simulink model "Simulink_file_newversion"  (R2024a)
settings: Solver=VariableStepAuto  StartTime=0.0  StopTime=5  RelTol=1e-3
values from neighbouring files (symbols this model uses):
  DG = cell(1, numOfDGs)    [evaluateDesigns.m]
  K = cell(1, numDGs)    [Centralized_Controller_For_DG.m]    (also in Centralized_Controller_For_DG_with_Constraints.m; ComputePassivityForDGs.m = sdpvar(1, 3, 'full'); GetPassivityForDGs.m = sdpvar(1, 3, 'full'); Global_Controller_Synthesis.m = cell(N, N))
  Line = cell(1, numOfLines)    [evaluateDesigns.m]
  V_ref = 48    [Global_Controller_Synthesis.m]
undefined symbols (not defined in the file or in its folder): ChangeGlobalLoad1, ChangeGlobalLoad2, PlugIn, PlugOut, R_Global, V_nom
libraries: spsSeriesRLCBranchLib x26, spsCurrentMeasurementLib x8, spsVoltageMeasurementLib x5, simulink x4, spsDCVoltageSourceLib x4, spsDiodeLib x4, spsIGBTLib x4, spsIdealSwitchLib x2, spsStairGeneratorLib x2, spspowerguiLib x1
settings Model: Creator=najaf  LastModifiedBy=najaf
settings RTWCC: GPUComputeCapability=3.5

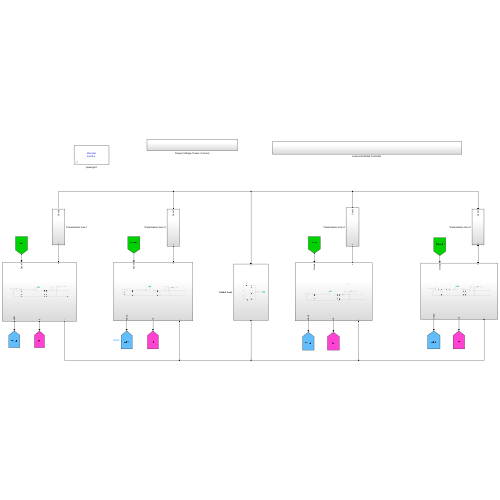
[thumbnail: Simulink's stored preview of the top-level diagram]
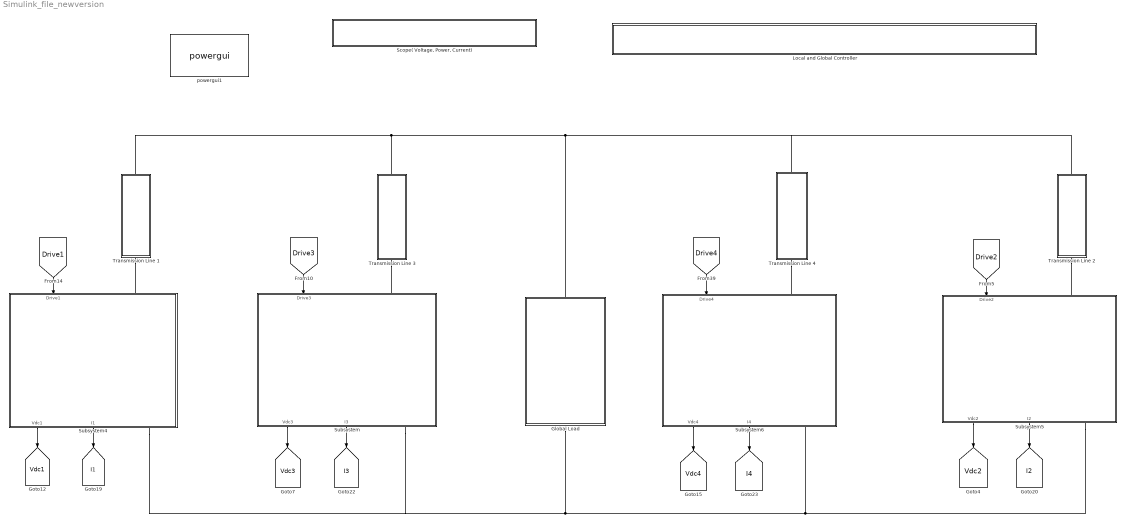
== system Simulink_file_newversion ==
  Global Load : Subsystem
  "Local and Global Controller " : Subsystem
  "Scope( Voltage, Power, Current)" : Subsystem
  Subsystem : Subsystem
      settings: PortSchema="{\"entries\":[{\"content\":{\"sides\":[{\"content\":{},\"type\":\"ConnectorPlacement.EquallySpacedRectSide\",\"uuid\":\"08b51d35-5d4f-4d5f-a5b0-37344ba45088\"},{\"content\":{\"side\":\"RIGHT\"},\"type\":\"ConnectorPlacement.EquallySpacedRectSide\",\"uuid\":\"3324977a-6e34-487c-ade0-88e1bff4bebb\"},{\"content\":{\"connectorIds\":[\"In1\",\"LConn1\"],\"side\":\"TOP\"},\"type\":\"ConnectorPlacement.EquallySpacedRectSide\",\"uuid\":\"e322db0d-0a35-4471-b922-f546e4cab97b\"},{\"content\":{\"connectorIds\":[\"Out1\",\"Out2\",\"RConn1\"],\"side\":\"BOTTOM\"},\"type\":\"ConnectorPlacement.EquallySpacedRectSide\",\"uuid\":\"57a428a6-4844-4d68-bda7-c5e0dfb814f7\"}]},\"type\":\"ConnectorPlacement.EquallySpacedConnector\",\"uuid\":\"93cb8cb8-3b8c-4430-b1f3-cf7722d9fa22\"}],\"packageUris\":[\"http://schema.mathworks.com/mf0/Connector/R2020b\"],\"version\":\"1.0\"}"
  Subsystem4 : Subsystem
      settings: PortSchema="{\"entries\":[{\"content\":{\"sides\":[{\"content\":{},\"type\":\"ConnectorPlacement.EquallySpacedRectSide\",\"uuid\":\"764b3ce9-8ebc-4171-9263-333df0dfe6fc\"},{\"content\":{\"side\":\"RIGHT\"},\"type\":\"ConnectorPlacement.EquallySpacedRectSide\",\"uuid\":\"c1e9d8a4-dae3-47b0-883a-539aeb69869c\"},{\"content\":{\"connectorIds\":[\"In1\",\"LConn1\"],\"side\":\"TOP\"},\"type\":\"ConnectorPlacement.EquallySpacedRectSide\",\"uuid\":\"bcad0197-72c7-4543-a9ab-ea7942b9cd59\"},{\"content\":{\"connectorIds\":[\"Out1\",\"Out2\",\"RConn1\"],\"side\":\"BOTTOM\"},\"type\":\"ConnectorPlacement.EquallySpacedRectSide\",\"uuid\":\"beb0f75b-103e-4e06-b52f-abd8ae36630a\"}]},\"type\":\"ConnectorPlacement.EquallySpacedConnector\",\"uuid\":\"3998def4-aed0-48b8-bc2a-5ab2d5ec9fd3\"}],\"packageUris\":[\"http://schema.mathworks.com/mf0/Connector/R2020b\"],\"version\":\"1.0\"}"
  Subsystem5 : Subsystem
      settings: PortSchema="{\"entries\":[{\"content\":{\"sides\":[{\"content\":{},\"type\":\"ConnectorPlacement.EquallySpacedRectSide\",\"uuid\":\"08b51d35-5d4f-4d5f-a5b0-37344ba45088\"},{\"content\":{\"side\":\"RIGHT\"},\"type\":\"ConnectorPlacement.EquallySpacedRectSide\",\"uuid\":\"3324977a-6e34-487c-ade0-88e1bff4bebb\"},{\"content\":{\"connectorIds\":[\"In1\",\"LConn1\"],\"side\":\"TOP\"},\"type\":\"ConnectorPlacement.EquallySpacedRectSide\",\"uuid\":\"e322db0d-0a35-4471-b922-f546e4cab97b\"},{\"content\":{\"connectorIds\":[\"Out1\",\"Out2\",\"RConn1\"],\"side\":\"BOTTOM\"},\"type\":\"ConnectorPlacement.EquallySpacedRectSide\",\"uuid\":\"f52eba1b-ac2a-4c74-a10c-8b92ab05ae45\"}]},\"type\":\"ConnectorPlacement.EquallySpacedConnector\",\"uuid\":\"93cb8cb8-3b8c-4430-b1f3-cf7722d9fa22\"}],\"packageUris\":[\"http://schema.mathworks.com/mf0/Connector/R2020b\"],\"version\":\"1.0\"}"
  Subsystem6 : Subsystem
      settings: PortSchema="{\"entries\":[{\"content\":{\"sides\":[{\"content\":{},\"type\":\"ConnectorPlacement.EquallySpacedRectSide\",\"uuid\":\"764b3ce9-8ebc-4171-9263-333df0dfe6fc\"},{\"content\":{\"side\":\"RIGHT\"},\"type\":\"ConnectorPlacement.EquallySpacedRectSide\",\"uuid\":\"c1e9d8a4-dae3-47b0-883a-539aeb69869c\"},{\"content\":{\"connectorIds\":[\"In1\",\"LConn1\"],\"side\":\"TOP\"},\"type\":\"ConnectorPlacement.EquallySpacedRectSide\",\"uuid\":\"bcad0197-72c7-4543-a9ab-ea7942b9cd59\"},{\"content\":{\"connectorIds\":[\"Out1\",\"Out2\",\"RConn1\"],\"side\":\"BOTTOM\"},\"type\":\"ConnectorPlacement.EquallySpacedRectSide\",\"uuid\":\"43195860-d6e2-4bd9-a504-1cc2264ea7f4\"}]},\"type\":\"ConnectorPlacement.EquallySpacedConnector\",\"uuid\":\"3998def4-aed0-48b8-bc2a-5ab2d5ec9fd3\"}],\"packageUris\":[\"http://schema.mathworks.com/mf0/Connector/R2020b\"],\"version\":\"1.0\"}"
  Transmission Line 1 : Subsystem
  Transmission Line 2 : Subsystem
  Transmission Line 3 : Subsystem
  Transmission Line 4 : Subsystem
  powergui1 : spspowerguiLib/powergui  Priority=1  SimulationMode=Discrete  SampleTime=2e-5  frequency=60  Iterations=50  frequencyindice=0  Pbase=100e6  ErrMax=1e-4  UnitsV=kV  UnitsW=MW  buscounter=0  FunctionMessages=off  echomessages=off  EnableUseOfTLC=off  CurrentSourceSwitches=off  DisableSnubberDevices=off  DisableRonSwitches=off  DisableVfSwitches=off  DisplayEquations=off  AutomaticDiscreteSolvers=off  SolverType=Tustin/Backward Euler (TBE)  Interpol=off  ExternalGateDelay=off  methode=off  Ts=100  x0status=blocks  SPID=on  SwTol=0  HookPort=off  NonlinearTolerance=1e-4  nMaxIteration=100  ContinueOnMaxIteration=off  RestoreLinks=warning  ResistiveCurrentMeasurement=off  Frange=[0:2:500]  Ylog=off  Xlog=on  ShowGrid=off  save=off  variable=ZData  structure=0  ZoomFFT=off  StartTime=0.0  cycles=1  DisplayStyle=1  fundamental=60  FreqAxis=off  MaxFrequency=1000  frequencyindicesteady=1  RmsSteady=1  display=off
  tag scope: I1=global, I2=global, I3=global, I4=global, Vdc1=global, Vdc2=global, Vdc3=global, Vdc4=global
  wires:
  [Drive4] -> Subsystem6/1(Drive4)
  Subsystem6/1(Vdc4) -> [Vdc4]
  Subsystem6/2(I4) -> [I4]
  [Drive1] -> Subsystem4/1(Drive1)
  Subsystem4/1(Vdc1) -> [Vdc1]
  Subsystem4/2(I1) -> [I1]
  [Drive2] -> Subsystem5/1(Drive2)
  [Drive3] -> Subsystem/1(Drive3)
  Subsystem/2(I3) -> [I3]
  Subsystem/1(Vdc3) -> [Vdc3]
  Subsystem5/1(Vdc2) -> [Vdc2]
  Subsystem5/2(I2) -> [I2]
  connections:
  Transmission Line 1/LConn1 -- Subsystem4/LConn1
  Subsystem5/RConn1 -- Subsystem4/RConn1 -- Subsystem/RConn1 -- Global Load/RConn1 -- Subsystem6/RConn1
  Transmission Line 2/RConn1 -- Subsystem5/LConn1
  Transmission Line 3/RConn1 -- Subsystem/LConn1
  Transmission Line 4/RConn1 -- Subsystem6/LConn1
  Transmission Line 1/RConn1 -- Transmission Line 2/LConn1 -- Transmission Line 4/LConn1 -- Global Load/LConn1 -- Transmission Line 3/LConn1

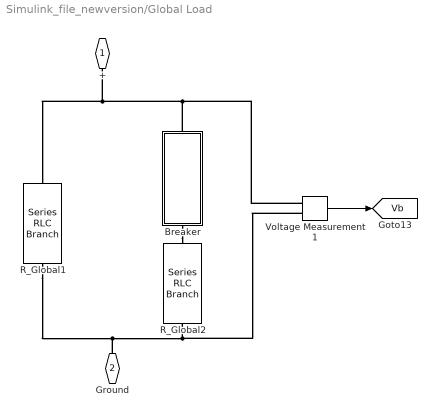
== system Simulink_file_newversion/Global Load ==
  Breaker : Subsystem
  R_Global1 : spsSeriesRLCBranchLib/Series RLC Branch  LConnTagsString=__new0  RConnTagsString=__new0  BranchType=R  Resistance=R_Global  Inductance=1e-3  SetiL0=off  InitialCurrent=0  Capacitance=1e-6  Setx0=off  InitialVoltage=0  Measurements=None
  R_Global2 : spsSeriesRLCBranchLib/Series RLC Branch  LConnTagsString=__new0  RConnTagsString=__new0  BranchType=R  Resistance=R_Global  Inductance=1e-3  SetiL0=off  InitialCurrent=0  Capacitance=1e-6  Setx0=off  InitialVoltage=0  Measurements=None
  Voltage Measurement1 : spsVoltageMeasurementLib/Voltage Measurement  PhasorSimulation=off  OutputType=Complex  PSBequivalent=0
  + : PMIOPort  Side=Left
  Ground : PMIOPort  Port=2  Side=Right
  tag scope: Vb=global
  wires:
  Voltage Measurement1/1 -> [Vb]
  connections:
  Ground/RConn1 -- Voltage Measurement1/LConn2 -- R_Global2/RConn1 -- R_Global1/RConn1
  Breaker/LConn1 -- R_Global1/LConn1 -- +/RConn1 -- Voltage Measurement1/LConn1
  Breaker/RConn1 -- R_Global2/LConn1

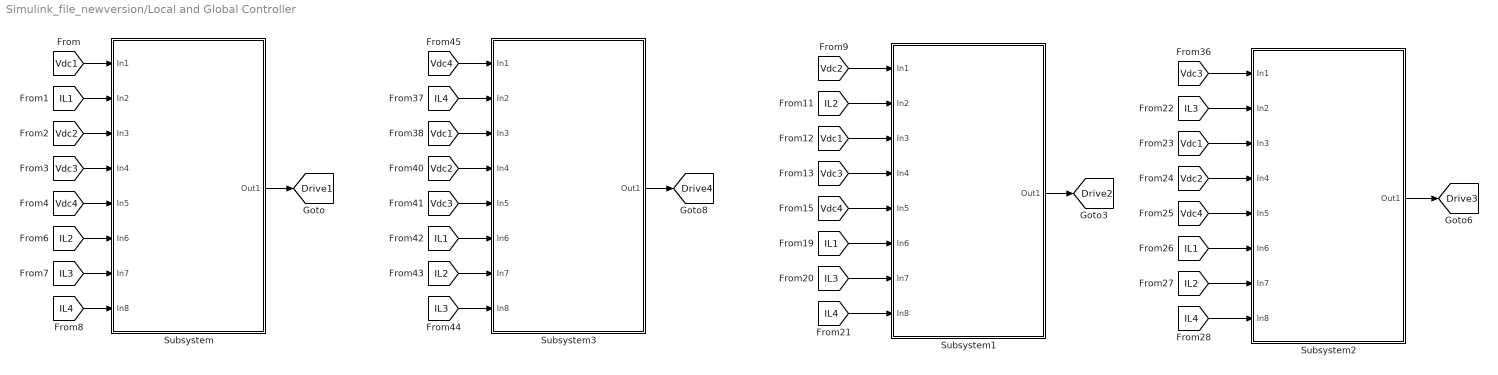
== system Simulink_file_newversion/Local and Global Controller  ==
  Subsystem : Subsystem
  Subsystem1 : Subsystem
  Subsystem2 : Subsystem
  Subsystem3 : Subsystem
  tag scope: Drive1=global, Drive2=global, Drive3=global, Drive4=global
  wires:
  [IL3] -> Subsystem3/8(In8)
  Subsystem3/1(Out1) -> [Drive4]
  [IL1] -> Subsystem3/6(In6)
  [IL2] -> Subsystem3/7(In7)
  [Vdc3] -> Subsystem1/4(In4)
  [IL4] -> Subsystem1/8(In8)
  [Vdc3] -> Subsystem3/5(In5)
  [IL4] -> Subsystem3/2(In2)
  [Vdc4] -> Subsystem3/1(In1)
  [Vdc1] -> Subsystem1/3(In3)
  [Vdc2] -> Subsystem3/4(In4)
  [Vdc1] -> Subsystem3/3(In3)
  [IL1] -> Subsystem1/6(In6)
  [Vdc4] -> Subsystem1/5(In5)
  [Vdc2] -> Subsystem1/1(In1)
  [IL3] -> Subsystem1/7(In7)
  Subsystem1/1(Out1) -> [Drive2]
  [IL2] -> Subsystem1/2(In2)
  Subsystem2/1(Out1) -> [Drive3]
  [IL3] -> Subsystem2/2(In2)
  [IL4] -> Subsystem2/8(In8)
  [Vdc2] -> Subsystem2/4(In4)
  [Vdc4] -> Subsystem2/5(In5)
  [IL1] -> Subsystem2/6(In6)
  [Vdc3] -> Subsystem2/1(In1)
  [Vdc1] -> Subsystem2/3(In3)
  [IL2] -> Subsystem2/7(In7)
  [Vdc2] -> Subsystem/3(In3)
  [Vdc4] -> Subsystem/5(In5)
  Subsystem/1(Out1) -> [Drive1]
  [IL2] -> Subsystem/6(In6)
  [IL3] -> Subsystem/7(In7)
  [IL4] -> Subsystem/8(In8)
  [IL1] -> Subsystem/2(In2)
  [Vdc1] -> Subsystem/1(In1)
  [Vdc3] -> Subsystem/4(In4)

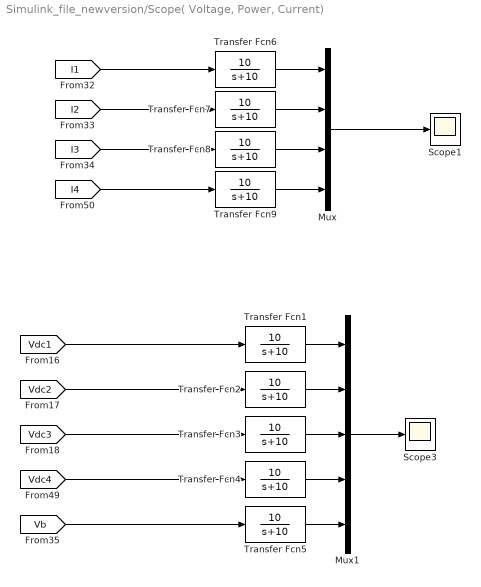
== system Simulink_file_newversion/Scope( Voltage, Power, Current) ==
  Mux : Mux
  Mux1 : Mux  Inputs=5
  Scope1 : Scope
  Scope3 : Scope
  Transfer Fcn{1..9} (9 alike) : TransferFcn  Numerator=[10]  Denominator=[1 10]
  wires:
  [I3] -> Transfer Fcn8/1
  [I2] -> Transfer Fcn7/1
  [I1] -> Transfer Fcn6/1
  Mux/1 -> Scope1/1
  [I4] -> Transfer Fcn9/1
  Mux1/1 -> Scope3/1
  [Vdc1] -> Transfer Fcn1/1
  [Vdc2] -> Transfer Fcn2/1
  [Vdc3] -> Transfer Fcn3/1
  [Vdc4] -> Transfer Fcn4/1
  [Vb] -> Transfer Fcn5/1
  Transfer Fcn1/1 -> Mux1/1
  Transfer Fcn2/1 -> Mux1/2
  Transfer Fcn3/1 -> Mux1/3
  Transfer Fcn4/1 -> Mux1/4
  Transfer Fcn5/1 -> Mux1/5
  Transfer Fcn6/1 -> Mux/1
  Transfer Fcn7/1 -> Mux/2
  Transfer Fcn8/1 -> Mux/3
  Transfer Fcn9/1 -> Mux/4

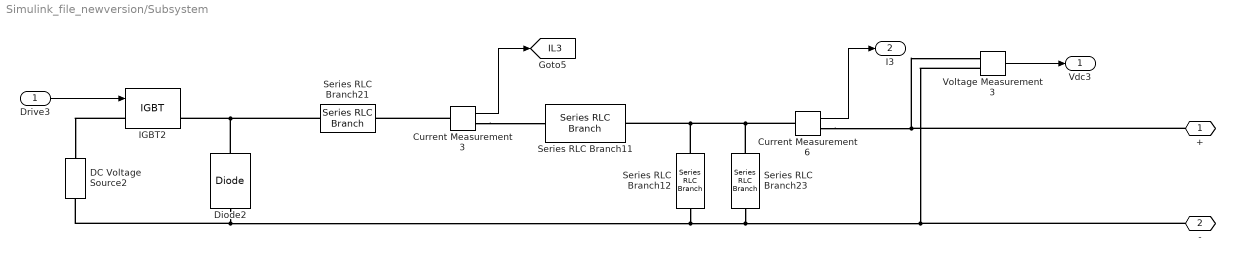
== system Simulink_file_newversion/Subsystem ==
  Drive3 : Inport
  Current Measurement3 : spsCurrentMeasurementLib/Current Measurement  PhasorSimulation=off  OutputType=Complex  PSBequivalent=0
  Current Measurement6 : spsCurrentMeasurementLib/Current Measurement  PhasorSimulation=off  OutputType=Complex  PSBequivalent=0
  DC Voltage Source2 : spsDCVoltageSourceLib/DC Voltage Source  Amplitude=V_nom  Measurements=None
  Diode2 : spsDiodeLib/Diode  Ron=0.001  Lon=0  Vf=0.8  IC=0  UseSnubber=off  Rs=500  Cs=0  Measurements=off
  IGBT2 : spsIGBTLib/IGBT  Ron=0.001  Lon=0  Vf=1  Tf=1e-6  Tt=2e-6  IC=0  Rs=1e5  Cs=inf  Measurements=on
  Series RLC Branch11 : spsSeriesRLCBranchLib/Series RLC Branch  LConnTagsString=__new0  RConnTagsString=__new0  BranchType=L  Resistance=1  Inductance=DG{3}.L  SetiL0=off  InitialCurrent=0  Capacitance=1e-6  Setx0=off  InitialVoltage=0  Measurements=Branch current
  Series RLC Branch12 : spsSeriesRLCBranchLib/Series RLC Branch  LConnTagsString=__new0  RConnTagsString=__new0  BranchType=C  Resistance=1  Inductance=1e-2  SetiL0=off  InitialCurrent=0  Capacitance=DG{3}.C  Setx0=off  InitialVoltage=0  Measurements=None
  Series RLC Branch21 : spsSeriesRLCBranchLib/Series RLC Branch  LConnTagsString=__new0  RConnTagsString=__new0  BranchType=R  Resistance=DG{3}.R  Inductance=1e-2  SetiL0=off  InitialCurrent=0  Capacitance=2.2e-3  Setx0=off  InitialVoltage=0  Measurements=None
  Series RLC Branch23 : spsSeriesRLCBranchLib/Series RLC Branch  LConnTagsString=__new0  RConnTagsString=__new0  BranchType=R  Resistance=DG{3}.Y  Inductance=1e-2  SetiL0=off  InitialCurrent=0  Capacitance=2.2e-3  Setx0=off  InitialVoltage=0  Measurements=None
  Voltage Measurement3 : spsVoltageMeasurementLib/Voltage Measurement  PhasorSimulation=off  OutputType=Complex  PSBequivalent=0
  + : PMIOPort  Side=Left
  - : PMIOPort  Port=2  Side=Right
  Vdc3 : Outport
  I3 : Outport  Port=2
  tag scope: IL3=global
  wires:
  Current Measurement3/1 -> [IL3]
  Drive3/1 -> IGBT2/1
  Current Measurement6/1 -> I3/1
  Voltage Measurement3/1 -> Vdc3/1
  connections:
  Series RLC Branch12/LConn1 -- Series RLC Branch23/LConn1 -- Current Measurement6/LConn1 -- Series RLC Branch11/RConn1
  Voltage Measurement3/LConn2 -- -/RConn1 -- Diode2/LConn1 -- DC Voltage Source2/LConn1 -- Series RLC Branch12/RConn1 -- Series RLC Branch23/RConn1
  Current Measurement6/RConn1 -- +/RConn1 -- Voltage Measurement3/LConn1
  Current Measurement3/LConn1 -- Series RLC Branch21/LConn1
  Current Measurement3/RConn1 -- Series RLC Branch11/LConn1
  Diode2/RConn1 -- Series RLC Branch21/RConn1 -- IGBT2/RConn1
  IGBT2/LConn1 -- DC Voltage Source2/RConn1

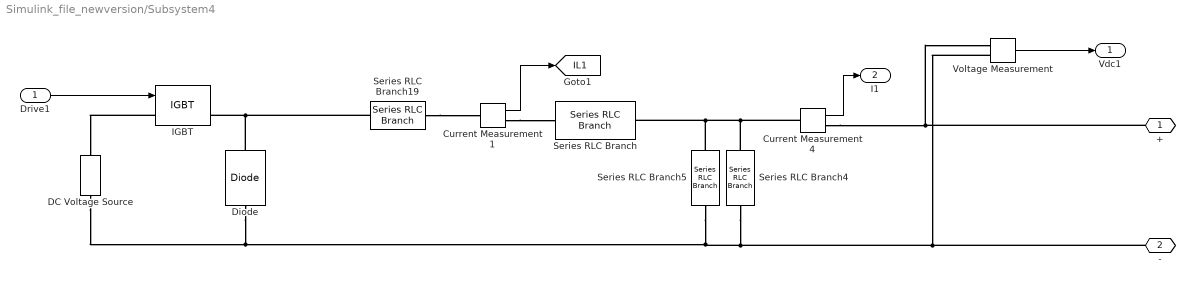
== system Simulink_file_newversion/Subsystem4 ==
  Drive1 : Inport
  Current Measurement1 : spsCurrentMeasurementLib/Current Measurement  PhasorSimulation=off  OutputType=Complex  PSBequivalent=0
  Current Measurement4 : spsCurrentMeasurementLib/Current Measurement  PhasorSimulation=off  OutputType=Complex  PSBequivalent=0
  DC Voltage Source : spsDCVoltageSourceLib/DC Voltage Source  Amplitude=V_nom  Measurements=None
  Diode : spsDiodeLib/Diode  Ron=0.001  Lon=0  Vf=0.8  IC=0  UseSnubber=off  Rs=500  Cs=0  Measurements=off
  IGBT : spsIGBTLib/IGBT  Ron=0.001  Lon=0  Vf=1  Tf=1e-6  Tt=2e-6  IC=0  Rs=1e5  Cs=inf  Measurements=on
  Series RLC Branch : spsSeriesRLCBranchLib/Series RLC Branch  LConnTagsString=__new0  RConnTagsString=__new0  BranchType=L  Resistance=1  Inductance=DG{1}.L  SetiL0=off  InitialCurrent=0  Capacitance=1e-6  Setx0=off  InitialVoltage=0  Measurements=Branch current
  Series RLC Branch19 : spsSeriesRLCBranchLib/Series RLC Branch  LConnTagsString=__new0  RConnTagsString=__new0  BranchType=R  Resistance=DG{1}.R  Inductance=1e-2  SetiL0=off  InitialCurrent=0  Capacitance=2.2e-3  Setx0=off  InitialVoltage=0  Measurements=None
  Series RLC Branch4 : spsSeriesRLCBranchLib/Series RLC Branch  LConnTagsString=__new0  RConnTagsString=__new0  BranchType=R  Resistance=DG{1}.Y  Inductance=1e-2  SetiL0=off  InitialCurrent=0  Capacitance=2.2e-3  Setx0=off  InitialVoltage=0  Measurements=None
  Series RLC Branch5 : spsSeriesRLCBranchLib/Series RLC Branch  LConnTagsString=__new0  RConnTagsString=__new0  BranchType=C  Resistance=1  Inductance=1e-2  SetiL0=off  InitialCurrent=0  Capacitance=DG{1}.C  Setx0=off  InitialVoltage=0  Measurements=None
  Voltage Measurement : spsVoltageMeasurementLib/Voltage Measurement  PhasorSimulation=off  OutputType=Complex  PSBequivalent=0
  + : PMIOPort  Side=Left
  - : PMIOPort  Port=2  Side=Right
  Vdc1 : Outport
  I1 : Outport  Port=2
  tag scope: IL1=global
  wires:
  Current Measurement1/1 -> [IL1]
  Current Measurement4/1 -> I1/1
  Voltage Measurement/1 -> Vdc1/1
  Drive1/1 -> IGBT/1
  connections:
  Current Measurement4/RConn1 -- +/RConn1 -- Voltage Measurement/LConn1
  Series RLC Branch4/RConn1 -- Voltage Measurement/LConn2 -- -/RConn1 -- DC Voltage Source/LConn1 -- Diode/LConn1 -- Series RLC Branch5/RConn1
  Series RLC Branch5/LConn1 -- Current Measurement4/LConn1 -- Series RLC Branch4/LConn1 -- Series RLC Branch/RConn1
  Current Measurement1/RConn1 -- Series RLC Branch/LConn1
  IGBT/LConn1 -- DC Voltage Source/RConn1
  Series RLC Branch19/LConn1 -- Current Measurement1/LConn1
  Diode/RConn1 -- Series RLC Branch19/RConn1 -- IGBT/RConn1

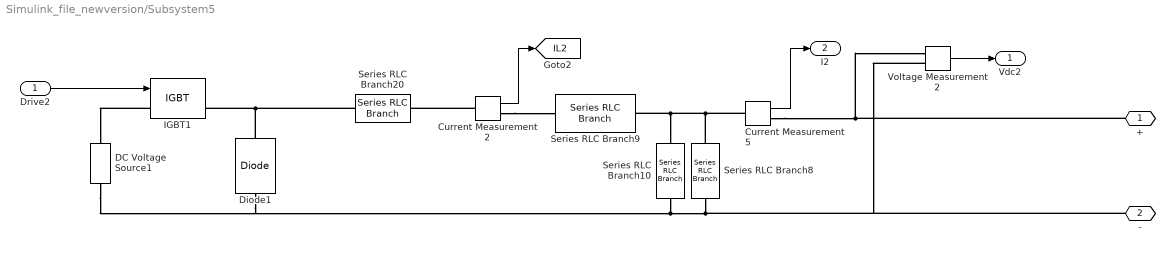
== system Simulink_file_newversion/Subsystem5 ==
  Drive2 : Inport
  Current Measurement2 : spsCurrentMeasurementLib/Current Measurement  PhasorSimulation=off  OutputType=Complex  PSBequivalent=0
  Current Measurement5 : spsCurrentMeasurementLib/Current Measurement  PhasorSimulation=off  OutputType=Complex  PSBequivalent=0
  DC Voltage Source1 : spsDCVoltageSourceLib/DC Voltage Source  Amplitude=V_nom  Measurements=None
  Diode1 : spsDiodeLib/Diode  Ron=0.001  Lon=0  Vf=0.8  IC=0  UseSnubber=off  Rs=500  Cs=0  Measurements=off
  IGBT1 : spsIGBTLib/IGBT  Ron=0.001  Lon=0  Vf=1  Tf=1e-6  Tt=2e-6  IC=0  Rs=1e5  Cs=inf  Measurements=on
  Series RLC Branch10 : spsSeriesRLCBranchLib/Series RLC Branch  LConnTagsString=__new0  RConnTagsString=__new0  BranchType=C  Resistance=1  Inductance=1e-2  SetiL0=off  InitialCurrent=0  Capacitance=DG{2}.C  Setx0=off  InitialVoltage=0  Measurements=None
  Series RLC Branch20 : spsSeriesRLCBranchLib/Series RLC Branch  LConnTagsString=__new0  RConnTagsString=__new0  BranchType=R  Resistance=DG{2}.R  Inductance=1e-2  SetiL0=off  InitialCurrent=0  Capacitance=2.2e-3  Setx0=off  InitialVoltage=0  Measurements=None
  Series RLC Branch8 : spsSeriesRLCBranchLib/Series RLC Branch  LConnTagsString=__new0  RConnTagsString=__new0  BranchType=R  Resistance=DG{2}.Y  Inductance=1e-2  SetiL0=off  InitialCurrent=0  Capacitance=2.2e-3  Setx0=off  InitialVoltage=0  Measurements=None
  Series RLC Branch9 : spsSeriesRLCBranchLib/Series RLC Branch  LConnTagsString=__new0  RConnTagsString=__new0  BranchType=L  Resistance=1  Inductance=DG{2}.L  SetiL0=off  InitialCurrent=0  Capacitance=1e-6  Setx0=off  InitialVoltage=0  Measurements=Branch current
  Voltage Measurement2 : spsVoltageMeasurementLib/Voltage Measurement  PhasorSimulation=off  OutputType=Complex  PSBequivalent=0
  + : PMIOPort  Side=Left
  - : PMIOPort  Port=2  Side=Right
  Vdc2 : Outport
  I2 : Outport  Port=2
  tag scope: IL2=global
  wires:
  Current Measurement2/1 -> [IL2]
  Drive2/1 -> IGBT1/1
  Current Measurement5/1 -> I2/1
  Voltage Measurement2/1 -> Vdc2/1
  connections:
  Series RLC Branch8/LConn1 -- Current Measurement5/LConn1 -- Series RLC Branch10/LConn1 -- Series RLC Branch9/RConn1
  Current Measurement5/RConn1 -- +/RConn1 -- Voltage Measurement2/LConn1
  Diode1/RConn1 -- Series RLC Branch20/RConn1 -- IGBT1/RConn1
  Series RLC Branch10/RConn1 -- DC Voltage Source1/LConn1 -- Diode1/LConn1 -- Voltage Measurement2/LConn2 -- -/RConn1 -- Series RLC Branch8/RConn1
  Current Measurement2/RConn1 -- Series RLC Branch9/LConn1
  Current Measurement2/LConn1 -- Series RLC Branch20/LConn1
  IGBT1/LConn1 -- DC Voltage Source1/RConn1

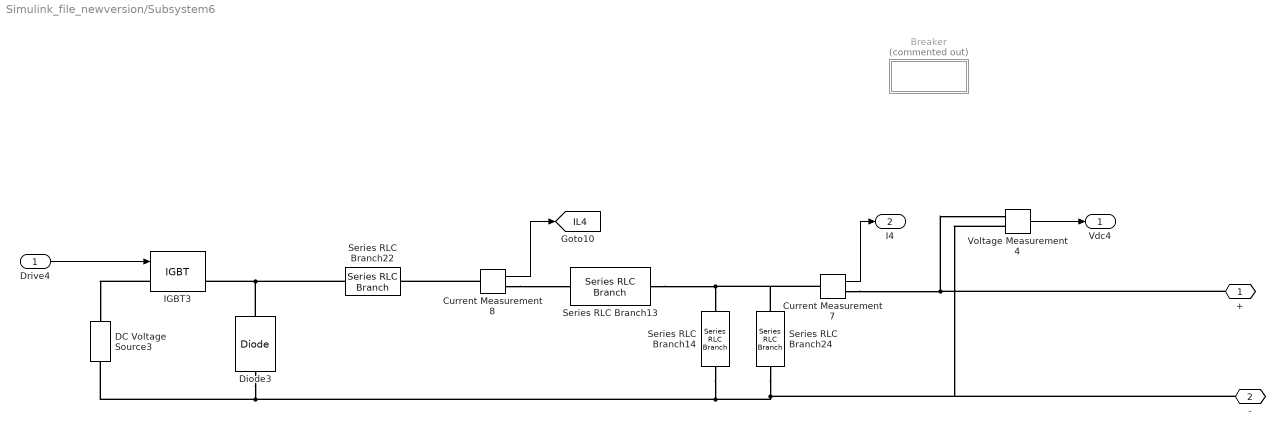
== system Simulink_file_newversion/Subsystem6 ==
  Drive4 : Inport
  Breaker : Subsystem  Commented=on
  Current Measurement7 : spsCurrentMeasurementLib/Current Measurement  PhasorSimulation=off  OutputType=Complex  PSBequivalent=0
  Current Measurement8 : spsCurrentMeasurementLib/Current Measurement  PhasorSimulation=off  OutputType=Complex  PSBequivalent=0
  DC Voltage Source3 : spsDCVoltageSourceLib/DC Voltage Source  Amplitude=V_nom  Measurements=None
  Diode3 : spsDiodeLib/Diode  Ron=0.001  Lon=0  Vf=0.8  IC=0  UseSnubber=off  Rs=500  Cs=0  Measurements=off
  IGBT3 : spsIGBTLib/IGBT  Ron=0.001  Lon=0  Vf=1  Tf=1e-6  Tt=2e-6  IC=0  Rs=1e5  Cs=inf  Measurements=on
  Series RLC Branch13 : spsSeriesRLCBranchLib/Series RLC Branch  LConnTagsString=__new0  RConnTagsString=__new0  BranchType=L  Resistance=1  Inductance=DG{4}.L  SetiL0=off  InitialCurrent=0  Capacitance=1e-6  Setx0=off  InitialVoltage=0  Measurements=Branch current
  Series RLC Branch14 : spsSeriesRLCBranchLib/Series RLC Branch  LConnTagsString=__new0  RConnTagsString=__new0  BranchType=C  Resistance=1  Inductance=1e-2  SetiL0=off  InitialCurrent=0  Capacitance=DG{4}.C  Setx0=off  InitialVoltage=0  Measurements=None
  Series RLC Branch22 : spsSeriesRLCBranchLib/Series RLC Branch  LConnTagsString=__new0  RConnTagsString=__new0  BranchType=R  Resistance=DG{4}.R  Inductance=1e-2  SetiL0=off  InitialCurrent=0  Capacitance=2.2e-3  Setx0=off  InitialVoltage=0  Measurements=None
  Series RLC Branch24 : spsSeriesRLCBranchLib/Series RLC Branch  LConnTagsString=__new0  RConnTagsString=__new0  BranchType=R  Resistance=DG{4}.Y  Inductance=1e-2  SetiL0=off  InitialCurrent=0  Capacitance=2.2e-3  Setx0=off  InitialVoltage=0  Measurements=None
  Voltage Measurement4 : spsVoltageMeasurementLib/Voltage Measurement  PhasorSimulation=off  OutputType=Complex  PSBequivalent=0
  + : PMIOPort  Side=Left
  - : PMIOPort  Port=2  Side=Right
  Vdc4 : Outport
  I4 : Outport  Port=2
  tag scope: IL4=global
  wires:
  Current Measurement8/1 -> [IL4]
  Current Measurement7/1 -> I4/1
  Voltage Measurement4/1 -> Vdc4/1
  Drive4/1 -> IGBT3/1
  connections:
  Series RLC Branch13/RConn1 -- Current Measurement7/LConn1 -- Series RLC Branch24/LConn1 -- Series RLC Branch14/LConn1
  Series RLC Branch14/RConn1 -- Voltage Measurement4/LConn2 -- -/RConn1 -- Series RLC Branch24/RConn1 -- Diode3/LConn1 -- DC Voltage Source3/LConn1
  IGBT3/LConn1 -- DC Voltage Source3/RConn1
  Current Measurement7/RConn1 -- +/RConn1 -- Voltage Measurement4/LConn1
  Diode3/RConn1 -- Series RLC Branch22/RConn1 -- IGBT3/RConn1
  Current Measurement8/LConn1 -- Series RLC Branch22/LConn1
  Current Measurement8/RConn1 -- Series RLC Branch13/LConn1

== system Simulink_file_newversion/Transmission Line 1 ==
  Series RLC Branch15 : spsSeriesRLCBranchLib/Series RLC Branch  LConnTagsString=__new0  RConnTagsString=__new0  BranchType=L  Resistance=1  Inductance=Line{1}.L  SetiL0=off  InitialCurrent=0  Capacitance=1e-6  Setx0=off  InitialVoltage=0  Measurements=Branch current
  Series RLC Branch6 : spsSeriesRLCBranchLib/Series RLC Branch  LConnTagsString=__new0  RConnTagsString=__new0  BranchType=R  Resistance=Line{1}.R  Inductance=1e-2  SetiL0=off  InitialCurrent=0  Capacitance=2.2e-3  Setx0=off  InitialVoltage=0  Measurements=None
  + : PMIOPort  Side=Left
  Conn2 : PMIOPort  Port=2  Side=Right
  connections:
  Series RLC Branch6/RConn1 -- +/RConn1
  Series RLC Branch15/LConn1 -- Series RLC Branch6/LConn1
  Series RLC Branch15/RConn1 -- Conn2/RConn1

== system Simulink_file_newversion/Transmission Line 2 ==
  Series RLC Branch1 : spsSeriesRLCBranchLib/Series RLC Branch  LConnTagsString=__new0  RConnTagsString=__new0  BranchType=R  Resistance=Line{2}.R  Inductance=1e-2  SetiL0=off  InitialCurrent=0  Capacitance=2.2e-3  Setx0=off  InitialVoltage=0  Measurements=None
  Series RLC Branch16 : spsSeriesRLCBranchLib/Series RLC Branch  LConnTagsString=__new0  RConnTagsString=__new0  BranchType=L  Resistance=1  Inductance=Line{2}.L  SetiL0=off  InitialCurrent=0  Capacitance=1e-6  Setx0=off  InitialVoltage=0  Measurements=Branch current
  Conn1 : PMIOPort  Side=Left
  + : PMIOPort  Port=2  Side=Right
  connections:
  Series RLC Branch16/LConn1 -- Series RLC Branch1/LConn1
  Series RLC Branch1/RConn1 -- Conn1/RConn1
  Series RLC Branch16/RConn1 -- +/RConn1

== system Simulink_file_newversion/Transmission Line 3 ==
  Series RLC Branch17 : spsSeriesRLCBranchLib/Series RLC Branch  LConnTagsString=__new0  RConnTagsString=__new0  BranchType=L  Resistance=1  Inductance=Line{3}.L  SetiL0=off  InitialCurrent=0  Capacitance=1e-6  Setx0=off  InitialVoltage=0  Measurements=Branch current
  Series RLC Branch2 : spsSeriesRLCBranchLib/Series RLC Branch  LConnTagsString=__new0  RConnTagsString=__new0  BranchType=R  Resistance=Line{3}.R  Inductance=1e-2  SetiL0=off  InitialCurrent=0  Capacitance=2.2e-3  Setx0=off  InitialVoltage=0  Measurements=None
  Conn1 : PMIOPort  Side=Left
  + : PMIOPort  Port=2  Side=Right
  connections:
  Series RLC Branch17/LConn1 -- Series RLC Branch2/LConn1
  Series RLC Branch2/RConn1 -- Conn1/RConn1
  Series RLC Branch17/RConn1 -- +/RConn1

== system Simulink_file_newversion/Transmission Line 4 ==
  Series RLC Branch18 : spsSeriesRLCBranchLib/Series RLC Branch  LConnTagsString=__new0  RConnTagsString=__new0  BranchType=L  Resistance=1  Inductance=Line{4}.L  SetiL0=off  InitialCurrent=0  Capacitance=1e-6  Setx0=off  InitialVoltage=0  Measurements=Branch current
  Series RLC Branch3 : spsSeriesRLCBranchLib/Series RLC Branch  LConnTagsString=__new0  RConnTagsString=__new0  BranchType=R  Resistance=Line{4}.R  Inductance=1e-2  SetiL0=off  InitialCurrent=0  Capacitance=2.2e-3  Setx0=off  InitialVoltage=0  Measurements=None
  Conn1 : PMIOPort  Side=Left
  + : PMIOPort  Port=2  Side=Right
  connections:
  Series RLC Branch18/LConn1 -- Series RLC Branch3/LConn1
  Series RLC Branch3/RConn1 -- Conn1/RConn1
  Series RLC Branch18/RConn1 -- +/RConn1

== system Simulink_file_newversion/Global Load/Breaker ==
  Ideal Switch : spsIdealSwitchLib/Ideal Switch  Ron=0.001  Lon=0  IC=0  Rs=1e5  Cs=inf  Measurements=on
  Stair Generator : spsStairGeneratorLib/Stair Generator  t=[0,ChangeGlobalLoad1,ChangeGlobalLoad2]  e=[0,1,0]  Ts=0
  + : PMIOPort  Side=Left
  load : PMIOPort  Port=2  Side=Right
  wires:
  Stair Generator/1 -> Ideal Switch/1
  connections:
  Ideal Switch/LConn1 -- +/RConn1
  Ideal Switch/RConn1 -- load/RConn1

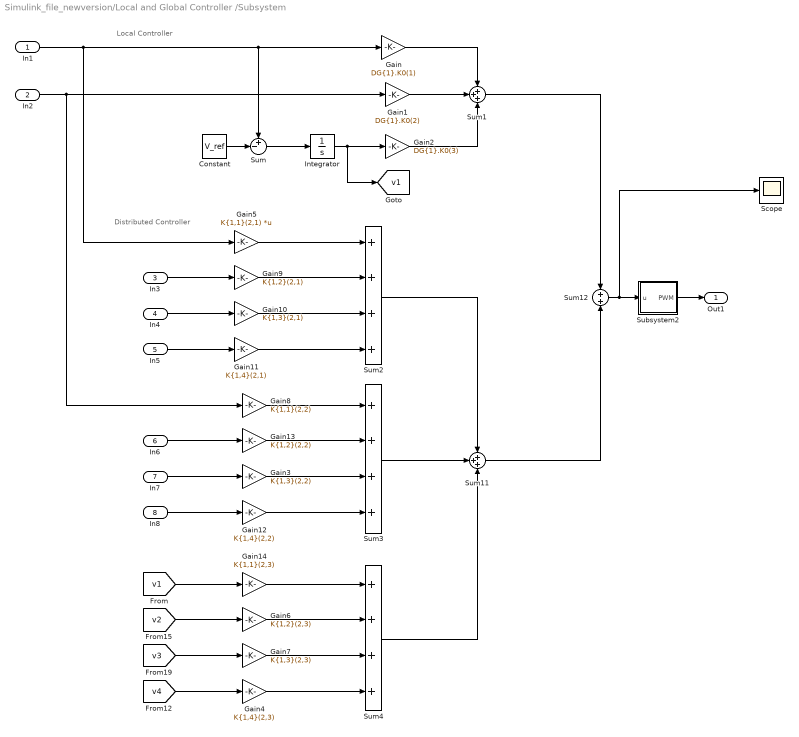
== system Simulink_file_newversion/Local and Global Controller /Subsystem ==
  note: Local Controller
  note: Distributed Controller
  In1 : Inport
  In2 : Inport  Port=2
  In3 : Inport  Port=3
  In4 : Inport  Port=4
  In5 : Inport  Port=5
  In6 : Inport  Port=6
  In7 : Inport  Port=7
  In8 : Inport  Port=8
  Constant : Constant  Value=V_ref
  Gain : Gain  Gain=DG{1}.K0(1)
  Gain1 : Gain  Gain=DG{1}.K0(2)
  Gain10 : Gain  Gain=K{1,3}(2,1)
  Gain11 : Gain  Gain=K{1,4}(2,1)
  Gain12 : Gain  Gain=K{1,4}(2,2)
  Gain13 : Gain  Gain=K{1,2}(2,2)
  Gain14 : Gain  Gain=K{1,1}(2,3)
  Gain2 : Gain  Gain=DG{1}.K0(3)
  Gain3 : Gain  Gain=K{1,3}(2,2)
  Gain4 : Gain  Gain=K{1,4}(2,3)
  Gain5 : Gain  Gain=K{1,1}(2,1)  Multiplication=Matrix(K*u)
  Gain6 : Gain  Gain=K{1,2}(2,3)
  Gain7 : Gain  Gain=K{1,3}(2,3)
  Gain8 : Gain  Gain=K{1,1}(2,2)
  Gain9 : Gain  Gain=K{1,2}(2,1)
  Integrator : Integrator
  Scope : Scope
  Subsystem2 : Subsystem
      mask Display: disp('PWM')
  Sum : Sum  Inputs=+-|
  Sum1 : Sum  Inputs=+++
  Sum11 : Sum  Inputs=+++
  Sum12 : Sum  Inputs=+|+
  Sum2 : Sum  Inputs=++++
  Sum3 : Sum  Inputs=++++
  Sum4 : Sum  Inputs=++++
  Out1 : Outport
  tag scope: v1=global
  wires:
  Sum12/1 -> Scope/1, Subsystem2/1(u)
  Gain/1 -> Sum1/1
  Constant/1 -> Sum/2
  Gain1/1 -> Sum1/2
  Sum1/1 -> Sum12/1
  Sum/1 -> Integrator/1
  Gain2/1 -> Sum1/3
  Gain6/1 -> Sum4/2
  Gain13/1 -> Sum3/2
  Gain12/1 -> Sum3/4
  Gain7/1 -> Sum4/3
  Gain5/1 -> Sum2/1
  Gain3/1 -> Sum3/3
  Sum11/1 -> Sum12/2
  Gain4/1 -> Sum4/4
  In4/1 -> Gain10/1
  [v3] -> Gain7/1
  In3/1 -> Gain9/1
  [v2] -> Gain6/1
  In6/1 -> Gain13/1
  [v4] -> Gain4/1
  In8/1 -> Gain12/1
  Gain10/1 -> Sum2/3
  In7/1 -> Gain3/1
  In5/1 -> Gain11/1
  Gain14/1 -> Sum4/1
  Gain11/1 -> Sum2/4
  Gain9/1 -> Sum2/2
  Gain8/1 -> Sum3/1
  [v1] -> Gain14/1
  Sum2/1 -> Sum11/1
  Sum3/1 -> Sum11/2
  Sum4/1 -> Sum11/3
  Integrator/1 -> [v1], Gain2/1
  In2/1 -> Gain1/1, Gain8/1
  In1/1 -> Gain/1, Sum/1, Gain5/1
  Subsystem2/1(PWM) -> Out1/1

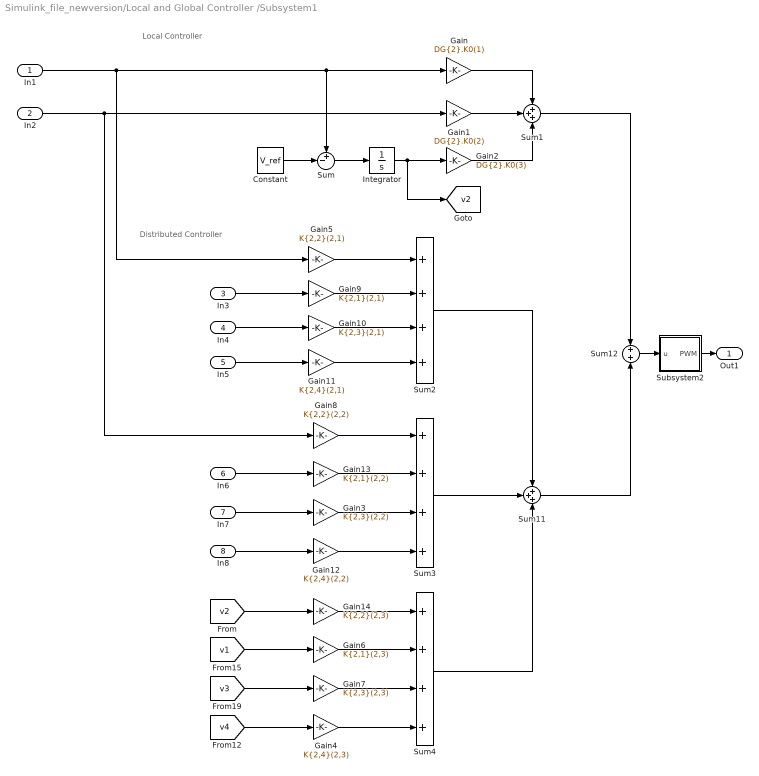
== system Simulink_file_newversion/Local and Global Controller /Subsystem1 ==
  note: Distributed Controller
  note: Local Controller
  In1 : Inport
  In2 : Inport  Port=2
  In3 : Inport  Port=3
  In4 : Inport  Port=4
  In5 : Inport  Port=5
  In6 : Inport  Port=6
  In7 : Inport  Port=7
  In8 : Inport  Port=8
  Constant : Constant  Value=V_ref
  Gain : Gain  Gain=DG{2}.K0(1)
  Gain1 : Gain  Gain=DG{2}.K0(2)
  Gain10 : Gain  Gain=K{2,3}(2,1)
  Gain11 : Gain  Gain=K{2,4}(2,1)
  Gain12 : Gain  Gain=K{2,4}(2,2)
  Gain13 : Gain  Gain=K{2,1}(2,2)
  Gain14 : Gain  Gain=K{2,2}(2,3)
  Gain2 : Gain  Gain=DG{2}.K0(3)
  Gain3 : Gain  Gain=K{2,3}(2,2)
  Gain4 : Gain  Gain=K{2,4}(2,3)
  Gain5 : Gain  Gain=K{2,2}(2,1)
  Gain6 : Gain  Gain=K{2,1}(2,3)
  Gain7 : Gain  Gain=K{2,3}(2,3)
  Gain8 : Gain  Gain=K{2,2}(2,2)
  Gain9 : Gain  Gain=K{2,1}(2,1)
  Integrator : Integrator
  Subsystem2 : Subsystem
      mask Display: disp('PWM')
  Sum : Sum  Inputs=+-|
  Sum1 : Sum  Inputs=+++
  Sum11 : Sum  Inputs=+++
  Sum12 : Sum  Inputs=+|+
  Sum2 : Sum  Inputs=++++
  Sum3 : Sum  Inputs=++++
  Sum4 : Sum  Inputs=++++
  Out1 : Outport
  tag scope: v2=global
  wires:
  Sum1/1 -> Sum12/1
  Gain1/1 -> Sum1/2
  Constant/1 -> Sum/2
  Gain/1 -> Sum1/1
  Gain2/1 -> Sum1/3
  Sum/1 -> Integrator/1
  In6/1 -> Gain13/1
  [v3] -> Gain7/1
  [v1] -> Gain6/1
  In4/1 -> Gain10/1
  In3/1 -> Gain9/1
  In5/1 -> Gain11/1
  In7/1 -> Gain3/1
  [v4] -> Gain4/1
  Sum11/1 -> Sum12/2
  In8/1 -> Gain12/1
  Gain5/1 -> Sum2/1
  Gain9/1 -> Sum2/2
  Gain10/1 -> Sum2/3
  Gain11/1 -> Sum2/4
  Gain8/1 -> Sum3/1
  Gain13/1 -> Sum3/2
  Gain3/1 -> Sum3/3
  Gain12/1 -> Sum3/4
  [v2] -> Gain14/1
  Gain14/1 -> Sum4/1
  Gain6/1 -> Sum4/2
  Gain7/1 -> Sum4/3
  Gain4/1 -> Sum4/4
  Sum2/1 -> Sum11/1
  Sum3/1 -> Sum11/2
  Sum4/1 -> Sum11/3
  Integrator/1 -> [v2], Gain2/1
  In2/1 -> Gain1/1, Gain8/1
  In1/1 -> Gain/1, Sum/1, Gain5/1
  Sum12/1 -> Subsystem2/1(u)
  Subsystem2/1(PWM) -> Out1/1

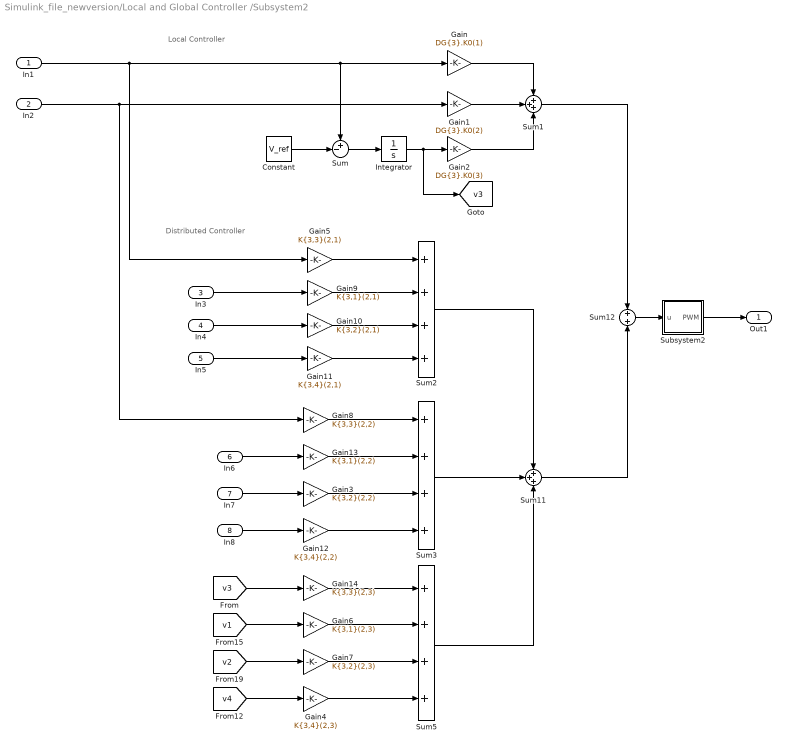
== system Simulink_file_newversion/Local and Global Controller /Subsystem2 ==
  note: Distributed Controller
  note: Local Controller
  In1 : Inport
  In2 : Inport  Port=2
  In3 : Inport  Port=3
  In4 : Inport  Port=4
  In5 : Inport  Port=5
  In6 : Inport  Port=6
  In7 : Inport  Port=7
  In8 : Inport  Port=8
  Constant : Constant  Value=V_ref
  Gain : Gain  Gain=DG{3}.K0(1)
  Gain1 : Gain  Gain=DG{3}.K0(2)
  Gain10 : Gain  Gain=K{3,2}(2,1)
  Gain11 : Gain  Gain=K{3,4}(2,1)
  Gain12 : Gain  Gain=K{3,4}(2,2)
  Gain13 : Gain  Gain=K{3,1}(2,2)
  Gain14 : Gain  Gain=K{3,3}(2,3)
  Gain2 : Gain  Gain=DG{3}.K0(3)
  Gain3 : Gain  Gain=K{3,2}(2,2)
  Gain4 : Gain  Gain=K{3,4}(2,3)
  Gain5 : Gain  Gain=K{3,3}(2,1)
  Gain6 : Gain  Gain=K{3,1}(2,3)
  Gain7 : Gain  Gain=K{3,2}(2,3)
  Gain8 : Gain  Gain=K{3,3}(2,2)
  Gain9 : Gain  Gain=K{3,1}(2,1)
  Integrator : Integrator
  Subsystem2 : Subsystem
      mask Display: disp('PWM')
  Sum : Sum  Inputs=+-|
  Sum1 : Sum  Inputs=+++
  Sum11 : Sum  Inputs=+++
  Sum12 : Sum  Inputs=+|+
  Sum2 : Sum  Inputs=++++
  Sum3 : Sum  Inputs=++++
  Sum5 : Sum  Inputs=++++
  Out1 : Outport
  tag scope: v3=global
  wires:
  Gain2/1 -> Sum1/3
  Gain/1 -> Sum1/1
  Constant/1 -> Sum/2
  Gain1/1 -> Sum1/2
  Sum1/1 -> Sum12/1
  Sum/1 -> Integrator/1
  Gain6/1 -> Sum5/2
  Gain13/1 -> Sum3/2
  Gain12/1 -> Sum3/4
  Gain7/1 -> Sum5/3
  Gain5/1 -> Sum2/1
  Gain3/1 -> Sum3/3
  Sum11/1 -> Sum12/2
  Gain4/1 -> Sum5/4
  In4/1 -> Gain10/1
  [v2] -> Gain7/1
  In3/1 -> Gain9/1
  [v1] -> Gain6/1
  In6/1 -> Gain13/1
  [v4] -> Gain4/1
  In8/1 -> Gain12/1
  Gain10/1 -> Sum2/3
  In7/1 -> Gain3/1
  In5/1 -> Gain11/1
  Gain14/1 -> Sum5/1
  Gain11/1 -> Sum2/4
  Gain9/1 -> Sum2/2
  Gain8/1 -> Sum3/1
  [v3] -> Gain14/1
  Sum2/1 -> Sum11/1
  Sum3/1 -> Sum11/2
  Sum5/1 -> Sum11/3
  Integrator/1 -> [v3], Gain2/1
  In2/1 -> Gain1/1, Gain8/1
  In1/1 -> Gain/1, Sum/1, Gain5/1
  Sum12/1 -> Subsystem2/1(u)
  Subsystem2/1(PWM) -> Out1/1

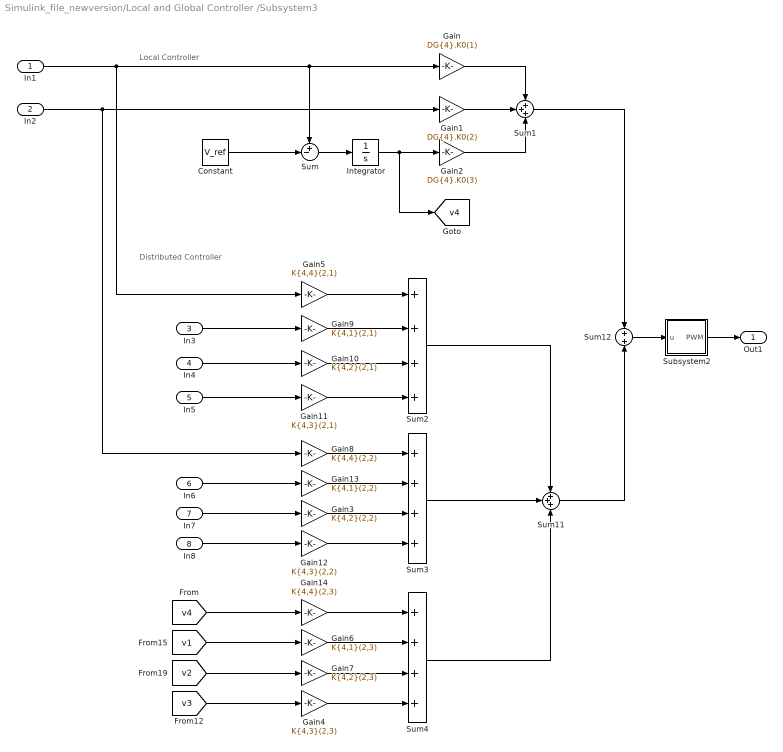
== system Simulink_file_newversion/Local and Global Controller /Subsystem3 ==
  note: Distributed Controller
  note: Local Controller
  In1 : Inport
  In2 : Inport  Port=2
  In3 : Inport  Port=3
  In4 : Inport  Port=4
  In5 : Inport  Port=5
  In6 : Inport  Port=6
  In7 : Inport  Port=7
  In8 : Inport  Port=8
  Constant : Constant  Value=V_ref
  Gain : Gain  Gain=DG{4}.K0(1)
  Gain1 : Gain  Gain=DG{4}.K0(2)
  Gain10 : Gain  Gain=K{4,2}(2,1)
  Gain11 : Gain  Gain=K{4,3}(2,1)
  Gain12 : Gain  Gain=K{4,3}(2,2)
  Gain13 : Gain  Gain=K{4,1}(2,2)
  Gain14 : Gain  Gain=K{4,4}(2,3)
  Gain2 : Gain  Gain=DG{4}.K0(3)
  Gain3 : Gain  Gain=K{4,2}(2,2)
  Gain4 : Gain  Gain=K{4,3}(2,3)
  Gain5 : Gain  Gain=K{4,4}(2,1)
  Gain6 : Gain  Gain=K{4,1}(2,3)
  Gain7 : Gain  Gain=K{4,2}(2,3)
  Gain8 : Gain  Gain=K{4,4}(2,2)
  Gain9 : Gain  Gain=K{4,1}(2,1)
  Integrator : Integrator
  Subsystem2 : Subsystem
      mask Display: disp('PWM')
  Sum : Sum  Inputs=+-|
  Sum1 : Sum  Inputs=+++
  Sum11 : Sum  Inputs=+++
  Sum12 : Sum  Inputs=+|+
  Sum2 : Sum  Inputs=++++
  Sum3 : Sum  Inputs=++++
  Sum4 : Sum  Inputs=++++
  Out1 : Outport
  tag scope: v4=global
  wires:
  Sum1/1 -> Sum12/1
  Gain1/1 -> Sum1/2
  Constant/1 -> Sum/2
  Gain/1 -> Sum1/1
  Gain2/1 -> Sum1/3
  Sum/1 -> Integrator/1
  Gain6/1 -> Sum4/2
  Gain13/1 -> Sum3/2
  Gain12/1 -> Sum3/4
  Gain7/1 -> Sum4/3
  Gain5/1 -> Sum2/1
  Gain3/1 -> Sum3/3
  Sum11/1 -> Sum12/2
  Gain4/1 -> Sum4/4
  In4/1 -> Gain10/1
  [v2] -> Gain7/1
  In3/1 -> Gain9/1
  [v1] -> Gain6/1
  In6/1 -> Gain13/1
  [v3] -> Gain4/1
  In8/1 -> Gain12/1
  Gain10/1 -> Sum2/3
  In7/1 -> Gain3/1
  In5/1 -> Gain11/1
  Gain14/1 -> Sum4/1
  Gain11/1 -> Sum2/4
  Gain9/1 -> Sum2/2
  Gain8/1 -> Sum3/1
  [v4] -> Gain14/1
  Sum2/1 -> Sum11/1
  Sum3/1 -> Sum11/2
  Sum4/1 -> Sum11/3
  Integrator/1 -> [v4], Gain2/1
  In2/1 -> Gain1/1, Gain8/1
  In1/1 -> Gain/1, Sum/1, Gain5/1
  Sum12/1 -> Subsystem2/1(u)
  Subsystem2/1(PWM) -> Out1/1

== system Simulink_file_newversion/Subsystem6/Breaker ==
  Ideal Switch : spsIdealSwitchLib/Ideal Switch  Ron=0.001  Lon=0  IC=0  Rs=1e5  Cs=inf  Measurements=on
  Stair Generator : spsStairGeneratorLib/Stair Generator  t=[0,PlugOut,PlugIn]  e=[1, 0, 1]  Ts=0
  DG4 : PMIOPort  Side=Left
  + : PMIOPort  Port=2  Side=Right
  wires:
  Stair Generator/1 -> Ideal Switch/1
  connections:
  Ideal Switch/LConn1 -- DG4/RConn1
  Ideal Switch/RConn1 -- +/RConn1

== system Simulink_file_newversion/Local and Global Controller /Subsystem/Subsystem2 ==
  u : Inport
  0.05 : Gain
  Relational Operator : RelationalOperator  OutDataTypeStr=boolean  InputSameDT=off
  Scope : Scope  NumInputPorts=2
  Scope2 : Scope
  Triangle1 : simulink/Sources/Repeating Sequence  rep_seq_t=[0 40e-5 80e-5]  rep_seq_y=[0 1 0]
  PWM : Outport
  wires:
  0.05/1 -> Relational Operator/1, Scope/1
  Triangle1/1 -> Relational Operator/2, Scope/2
  u/1 -> 0.05/1
  Relational Operator/1 -> PWM/1, Scope2/1

== system Simulink_file_newversion/Local and Global Controller /Subsystem1/Subsystem2 ==
  u : Inport
  0.05 : Gain
  Relational Operator : RelationalOperator  OutDataTypeStr=boolean  InputSameDT=off
  Scope : Scope  NumInputPorts=2
  Scope2 : Scope
  Triangle1 : simulink/Sources/Repeating Sequence  rep_seq_t=[0 40e-5 80e-5]  rep_seq_y=[0 1 0]
  PWM : Outport
  wires:
  0.05/1 -> Relational Operator/1, Scope/1
  Triangle1/1 -> Relational Operator/2, Scope/2
  u/1 -> 0.05/1
  Relational Operator/1 -> PWM/1, Scope2/1

== system Simulink_file_newversion/Local and Global Controller /Subsystem2/Subsystem2 ==
  u : Inport
  0.05 : Gain
  Relational Operator : RelationalOperator  OutDataTypeStr=boolean  InputSameDT=off
  Scope : Scope  NumInputPorts=2
  Scope2 : Scope
  Triangle1 : simulink/Sources/Repeating Sequence  rep_seq_t=[0 40e-5 80e-5]  rep_seq_y=[0 1 0]
  PWM : Outport
  wires:
  0.05/1 -> Relational Operator/1, Scope/1
  Triangle1/1 -> Relational Operator/2, Scope/2
  u/1 -> 0.05/1
  Relational Operator/1 -> PWM/1, Scope2/1

== system Simulink_file_newversion/Local and Global Controller /Subsystem3/Subsystem2 ==
  u : Inport
  0.05 : Gain
  Relational Operator : RelationalOperator  OutDataTypeStr=boolean  InputSameDT=off
  Scope : Scope  NumInputPorts=2
  Scope2 : Scope
  Triangle1 : simulink/Sources/Repeating Sequence  rep_seq_t=[0 40e-5 80e-5]  rep_seq_y=[0 1 0]
  PWM : Outport
  wires:
  0.05/1 -> Relational Operator/1, Scope/1
  Triangle1/1 -> Relational Operator/2, Scope/2
  u/1 -> 0.05/1
  Relational Operator/1 -> PWM/1, Scope2/1
